simulink model "evaluate_original_controller"  (R2020b)
settings: Solver=VariableStepAuto  StartTime=0.0  StopTime=100  RelTol=1e-3
settings Model: Creator=sharm  LastModifiedBy=Abhijit

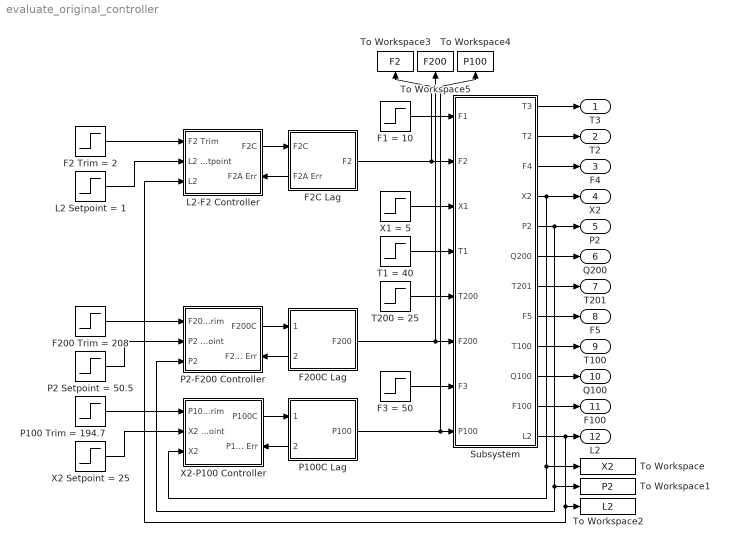
== system evaluate_original_controller ==
  F1 = 10 : Step  Time=0  After=10  SampleTime=0
  F2 Trim = 2 : Step  Time=0  After=2  SampleTime=0
  F200 Trim = 208 : Step  Time=0  After=208  SampleTime=0
  F200C Lag : Subsystem
      settings: PortSchema="{\"entries\":[{\"content\":{\"sides\":[{\"content\":{\"connectorIds\":[\"In1\",\"Out2\"]},\"type\":\"ConnectorPlacement.EquallySpacedRectSide\",\"uuid\":\"1c3b5bbe-eb64-4cf8-b304-9bf07220404b\"},{\"content\":{\"connectorIds\":[\"Out1\"],\"side\":\"RIGHT\"},\"type\":\"ConnectorPlacement.EquallySpacedRectSide\",\"uuid\":\"6c2af0ff-ea38-462b-984a-3066c6908657\"},{\"content\":{\"connectorIds\":[],\"side\":\"TOP\"},\"type\":\"ConnectorPlacement.EquallySpacedRectSide\",\"uuid\":\"8a7c128d-c093-40ae-be05-769f76d364e8\"},{\"content\":{\"connectorIds\":[],\"side\":\"HIDDEN\"},\"type\":\"ConnectorPlacement.EquallySpacedRectSide\",\"uuid\":\"6249208d-1a89-4983-a2d1-3ae1d70edd23\"}]},\"type\":\"ConnectorPlacement.EquallySpacedConnector\",\"uuid\":\"06c805ce-2383-4e6d-828b-e0ccee0563b2\"}],\"packageUris\":[\"http://schema.mathworks.com/mf0/Connector/R2020b\"],\"version\":\"1.0\"}"
  F2C Lag : Subsystem
      settings: PortSchema="{\"entries\":[{\"content\":{\"sides\":[{\"content\":{\"connectorIds\":[\"In1\",\"Out2\"]},\"type\":\"ConnectorPlacement.EquallySpacedRectSide\",\"uuid\":\"1c3b5bbe-eb64-4cf8-b304-9bf07220404b\"},{\"content\":{\"connectorIds\":[\"Out1\"],\"side\":\"RIGHT\"},\"type\":\"ConnectorPlacement.EquallySpacedRectSide\",\"uuid\":\"6c2af0ff-ea38-462b-984a-3066c6908657\"},{\"content\":{\"connectorIds\":[],\"side\":\"TOP\"},\"type\":\"ConnectorPlacement.EquallySpacedRectSide\",\"uuid\":\"8a7c128d-c093-40ae-be05-769f76d364e8\"},{\"content\":{\"connectorIds\":[],\"side\":\"HIDDEN\"},\"type\":\"ConnectorPlacement.EquallySpacedRectSide\",\"uuid\":\"6249208d-1a89-4983-a2d1-3ae1d70edd23\"}]},\"type\":\"ConnectorPlacement.EquallySpacedConnector\",\"uuid\":\"06c805ce-2383-4e6d-828b-e0ccee0563b2\"}],\"packageUris\":[\"http://schema.mathworks.com/mf0/Connector/R2020b\"],\"version\":\"1.0\"}"
  F3 = 50 : Step  Time=0  After=50  SampleTime=0
  L2 Setpoint = 1 : Step  Time=0  SampleTime=0
  L2-F2 Controller : Subsystem
      settings: PortSchema="{\"entries\":[{\"content\":{\"sides\":[{\"content\":{\"connectorIds\":[\"In1\",\"In2\",\"In3\"]},\"type\":\"ConnectorPlacement.EquallySpacedRectSide\",\"uuid\":\"ef4d4ad5-d901-40f4-ab80-7b76a95becde\"},{\"content\":{\"connectorIds\":[\"Out1\",\"In4\"],\"side\":\"RIGHT\"},\"type\":\"ConnectorPlacement.EquallySpacedRectSide\",\"uuid\":\"2e3077cf-f85a-4001-bdaf-12bb693cb162\"},{\"content\":{\"connectorIds\":[],\"side\":\"TOP\"},\"type\":\"ConnectorPlacement.EquallySpacedRectSide\",\"uuid\":\"9371a95a-1f33-4289-96cf-45c2d57bb552\"},{\"content\":{\"connectorIds\":[],\"side\":\"HIDDEN\"},\"type\":\"ConnectorPlacement.EquallySpacedRectSide\",\"uuid\":\"48f9f8fb-fea7-44ca-a8f8-23ec64a6d384\"}]},\"type\":\"ConnectorPlacement.EquallySpacedConnector\",\"uuid\":\"95306fdf-8f22-41f0-a056-501cc3b95527\"}],\"packageUris\":[\"http://schema.mathworks.com/mf0/Connector/R2020b\"],\"version\":\"1.0\"}"
  P100 Trim = 194.7 : Step  Time=0  After=194.7  SampleTime=0
  P100C Lag : Subsystem
      settings: PortSchema="{\"entries\":[{\"content\":{\"sides\":[{\"content\":{\"connectorIds\":[\"In1\",\"Out2\"]},\"type\":\"ConnectorPlacement.EquallySpacedRectSide\",\"uuid\":\"1c3b5bbe-eb64-4cf8-b304-9bf07220404b\"},{\"content\":{\"connectorIds\":[\"Out1\"],\"side\":\"RIGHT\"},\"type\":\"ConnectorPlacement.EquallySpacedRectSide\",\"uuid\":\"6c2af0ff-ea38-462b-984a-3066c6908657\"},{\"content\":{\"connectorIds\":[],\"side\":\"TOP\"},\"type\":\"ConnectorPlacement.EquallySpacedRectSide\",\"uuid\":\"8a7c128d-c093-40ae-be05-769f76d364e8\"},{\"content\":{\"connectorIds\":[],\"side\":\"HIDDEN\"},\"type\":\"ConnectorPlacement.EquallySpacedRectSide\",\"uuid\":\"6249208d-1a89-4983-a2d1-3ae1d70edd23\"}]},\"type\":\"ConnectorPlacement.EquallySpacedConnector\",\"uuid\":\"06c805ce-2383-4e6d-828b-e0ccee0563b2\"}],\"packageUris\":[\"http://schema.mathworks.com/mf0/Connector/R2020b\"],\"version\":\"1.0\"}"
  P2 Setpoint = 50.5 : Step  Time=0  After=50.5  SampleTime=0
  P2-F200 Controller : Subsystem
      settings: PortSchema="{\"entries\":[{\"content\":{\"sides\":[{\"content\":{\"connectorIds\":[\"In1\",\"In2\",\"In3\"]},\"type\":\"ConnectorPlacement.EquallySpacedRectSide\",\"uuid\":\"efbfbbac-d1e8-4a8e-b8ab-62373299654b\"},{\"content\":{\"connectorIds\":[\"Out1\",\"In4\"],\"side\":\"RIGHT\"},\"type\":\"ConnectorPlacement.EquallySpacedRectSide\",\"uuid\":\"c58e02ed-8699-419e-a739-83aeea4730ec\"},{\"content\":{\"connectorIds\":[],\"side\":\"TOP\"},\"type\":\"ConnectorPlacement.EquallySpacedRectSide\",\"uuid\":\"6be78c43-8237-4941-bb5c-cd018c1dcd72\"},{\"content\":{\"connectorIds\":[],\"side\":\"HIDDEN\"},\"type\":\"ConnectorPlacement.EquallySpacedRectSide\",\"uuid\":\"857e6460-9b7a-4c8b-b076-9e161e4e69bc\"}]},\"type\":\"ConnectorPlacement.EquallySpacedConnector\",\"uuid\":\"c2581144-7ad0-4f3d-846a-09b725ec330e\"}],\"packageUris\":[\"http://schema.mathworks.com/mf0/Connector/R2020b\"],\"version\":\"1.0\"}"
  Subsystem : Subsystem
  T1 = 40 : Step  Time=0  After=40  SampleTime=0
  T200 = 25 : Step  Time=0  After=25  SampleTime=0
  To Workspace : ToWorkspace  VariableName=X2  SaveFormat=Timeseries  SampleTime=-1
  To Workspace1 : ToWorkspace  VariableName=P2  SaveFormat=Timeseries  SampleTime=-1
  To Workspace2 : ToWorkspace  VariableName=L2  SaveFormat=Timeseries  SampleTime=-1
  To Workspace3 : ToWorkspace  VariableName=F2  SaveFormat=Timeseries  SampleTime=-1
  To Workspace4 : ToWorkspace  VariableName=P100  SaveFormat=Timeseries  SampleTime=-1
  To Workspace5 : ToWorkspace  VariableName=F200  SaveFormat=Timeseries  SampleTime=-1
  X1 = 5 : Step  Time=0  After=5  SampleTime=0
  X2 Setpoint = 25 : Step  Time=0  After=25  SampleTime=0
  X2-P100 Controller : Subsystem
      settings: PortSchema="{\"entries\":[{\"content\":{\"sides\":[{\"content\":{\"connectorIds\":[\"In1\",\"In2\",\"In3\"]},\"type\":\"ConnectorPlacement.EquallySpacedRectSide\",\"uuid\":\"5176dffd-dac1-4f9a-92a2-c3fec1393752\"},{\"content\":{\"connectorIds\":[\"Out1\",\"In4\"],\"side\":\"RIGHT\"},\"type\":\"ConnectorPlacement.EquallySpacedRectSide\",\"uuid\":\"ca0c7e9c-49dd-444e-80c7-5413a8e537a6\"},{\"content\":{\"connectorIds\":[],\"side\":\"TOP\"},\"type\":\"ConnectorPlacement.EquallySpacedRectSide\",\"uuid\":\"a41274ea-81fe-4467-9d67-a42c6c088fa1\"},{\"content\":{\"connectorIds\":[],\"side\":\"HIDDEN\"},\"type\":\"ConnectorPlacement.EquallySpacedRectSide\",\"uuid\":\"a4d67f8d-295f-4f62-a506-6c78b119ab3d\"}]},\"type\":\"ConnectorPlacement.EquallySpacedConnector\",\"uuid\":\"c27aa63c-44fb-4ea2-acae-9f89fa1a7cde\"}],\"packageUris\":[\"http://schema.mathworks.com/mf0/Connector/R2020b\"],\"version\":\"1.0\"}"
  T3 : Outport
  T2 : Outport  Port=2
  F4 : Outport  Port=3
  X2 : Outport  Port=4
  P2 : Outport  Port=5
  Q200 : Outport  Port=6
  T201 : Outport  Port=7
  F5 : Outport  Port=8
  T100 : Outport  Port=9
  Q100 : Outport  Port=10
  F100 : Outport  Port=11
  L2 : Outport  Port=12
  wires:
  F1 = 10/1 -> Subsystem/1(F1)
  X1 = 5/1 -> Subsystem/3(X1)
  T1 = 40/1 -> Subsystem/4(T1)
  T200 = 25/1 -> Subsystem/5(T200)
  F3 = 50/1 -> Subsystem/7(F3)
  Subsystem/1(T3) -> T3/1
  Subsystem/2(T2) -> T2/1
  Subsystem/3(F4) -> F4/1
  Subsystem/4(X2) -> X2-P100 Controller/3(X2), To Workspace/1, X2/1
  Subsystem/5(P2) -> P2/1, To Workspace1/1, P2-F200 Controller/3(P2)
  Subsystem/6(Q200) -> Q200/1
  Subsystem/7(T201) -> T201/1
  Subsystem/8(F5) -> F5/1
  Subsystem/9(T100) -> T100/1
  Subsystem/10(Q100) -> Q100/1
  Subsystem/11(F100) -> F100/1
  Subsystem/12(L2) -> L2/1, To Workspace2/1, L2-F2 Controller/3(L2)
  X2-P100 Controller/1(P100C) -> P100C Lag/1(P100C)
  P100C Lag/2(P100A Err) -> X2-P100 Controller/4(P100A Err)
  F200C Lag/2(F200A Err) -> P2-F200 Controller/4(F200A Err)
  P2-F200 Controller/1(F200C) -> F200C Lag/1(F200C)
  L2-F2 Controller/1(F2C) -> F2C Lag/1(F2C)
  F2C Lag/2(F2A Err) -> L2-F2 Controller/4(F2A Err)
  F200C Lag/1(F200) -> To Workspace5/1, Subsystem/6(F200)
  P100C Lag/1(P100) -> To Workspace4/1, Subsystem/8(P100)
  F2C Lag/1(F2) -> To Workspace3/1, Subsystem/2(F2)
  P2 Setpoint = 50.5/1 -> P2-F200 Controller/2(P2 Setpoint)
  L2 Setpoint = 1/1 -> L2-F2 Controller/2(L2 Setpoint)
  X2 Setpoint = 25/1 -> X2-P100 Controller/2(X2 Setpoint)
  P100 Trim = 194.7/1 -> X2-P100 Controller/1(P100 Trim)
  F2 Trim = 2/1 -> L2-F2 Controller/1(F2 Trim)
  F200 Trim = 208/1 -> P2-F200 Controller/1(F200 Trim)

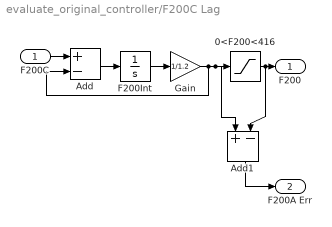
== system evaluate_original_controller/F200C Lag ==
  F200C : Inport
  0<F200<416 : Saturate  UpperLimit=416  LowerLimit=0
  Add : Sum  Inputs=+-
  Add1 : Sum  Inputs=+-
  F200Int : Integrator  InitialCondition=208
  Gain : Gain  Gain=1/1.2
  F200 : Outport
  F200A Err : Outport  Port=2
  wires:
  Gain/1 -> Add/2, Add1/1, 0<F200<416/1
  Add/1 -> F200Int/1
  F200Int/1 -> Gain/1
  F200C/1 -> Add/1
  0<F200<416/1 -> Add1/2, F200/1
  Add1/1 -> F200A Err/1

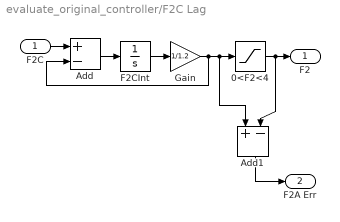
== system evaluate_original_controller/F2C Lag ==
  F2C : Inport
  0<F2<4 : Saturate  UpperLimit=4  LowerLimit=0
  Add : Sum  Inputs=+-
  Add1 : Sum  Inputs=+-
  F2CInt : Integrator  InitialCondition=2
  Gain : Gain  Gain=1/1.2
  F2 : Outport
  F2A Err : Outport  Port=2
  wires:
  Gain/1 -> Add/2, Add1/1, 0<F2<4/1
  Add/1 -> F2CInt/1
  F2CInt/1 -> Gain/1
  F2C/1 -> Add/1
  0<F2<4/1 -> Add1/2, F2/1
  Add1/1 -> F2A Err/1

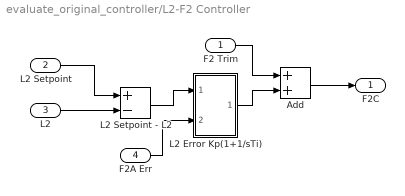
== system evaluate_original_controller/L2-F2 Controller ==
  F2 Trim : Inport
  L2 Setpoint : Inport  Port=2
  L2 : Inport  Port=3
  F2A Err : Inport  Port=4
  Add : Sum
  L2 Error Kp(1+1/sTi) : Subsystem
  L2 Setpoint - L2 : Sum  Inputs=+-
  F2C : Outport
  wires:
  L2 Setpoint/1 -> L2 Setpoint - L2/1
  F2 Trim/1 -> Add/1
  L2/1 -> L2 Setpoint - L2/2
  L2 Error Kp(1+1/sTi)/1(dF2C) -> Add/2
  L2 Setpoint - L2/1 -> L2 Error Kp(1+1/sTi)/1(F2 Err)
  Add/1 -> F2C/1
  F2A Err/1 -> L2 Error Kp(1+1/sTi)/2(F2A Err)

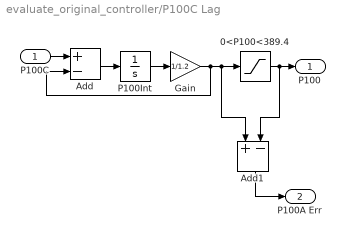
== system evaluate_original_controller/P100C Lag ==
  P100C : Inport
  0<P100<389.4 : Saturate  UpperLimit=389.4  LowerLimit=0
  Add : Sum  Inputs=+-
  Add1 : Sum  Inputs=+-
  Gain : Gain  Gain=1/1.2
  P100Int : Integrator  InitialCondition=194.7
  P100 : Outport
  P100A Err : Outport  Port=2
  wires:
  Gain/1 -> Add/2, 0<P100<389.4/1, Add1/1
  Add/1 -> P100Int/1
  P100Int/1 -> Gain/1
  P100C/1 -> Add/1
  0<P100<389.4/1 -> Add1/2, P100/1
  Add1/1 -> P100A Err/1

== system evaluate_original_controller/P2-F200 Controller ==
  F200 Trim : Inport
  P2 Setpoint : Inport  Port=2
  P2 : Inport  Port=3
  F200A Err : Inport  Port=4
  Add : Sum
  P2 Error Kp(1+1/sTi) : Subsystem
  P2 Setpoint - P2 : Sum  Inputs=+-
  F200C : Outport
  wires:
  P2 Setpoint/1 -> P2 Setpoint - P2/1
  F200 Trim/1 -> Add/1
  Add/1 -> F200C/1
  P2/1 -> P2 Setpoint - P2/2
  P2 Error Kp(1+1/sTi)/1(dF200C) -> Add/2
  P2 Setpoint - P2/1 -> P2 Error Kp(1+1/sTi)/1(P2 Err)
  F200A Err/1 -> P2 Error Kp(1+1/sTi)/2(F200A Err)

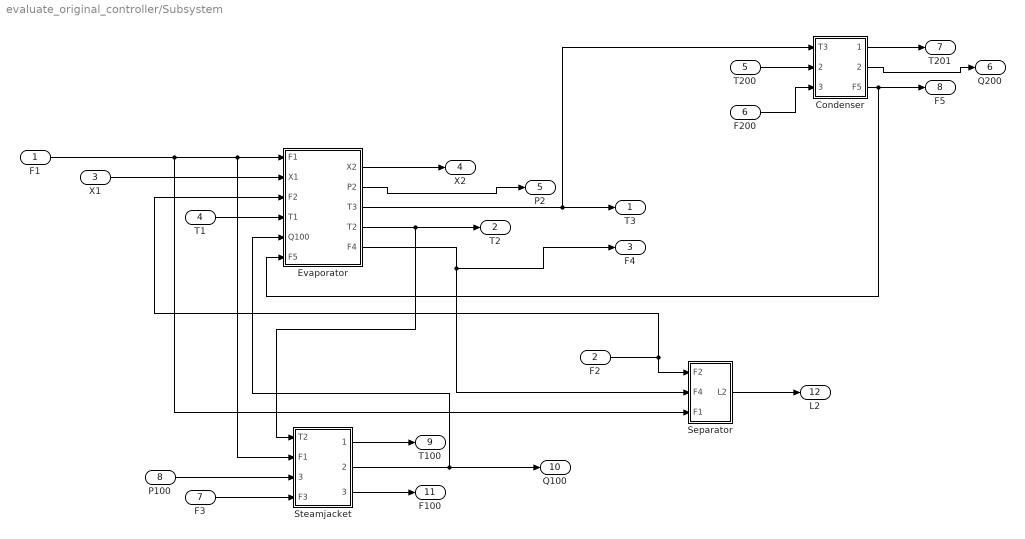
== system evaluate_original_controller/Subsystem ==
  F1 : Inport
  F2 : Inport  Port=2
  X1 : Inport  Port=3
  T1 : Inport  Port=4
  T200 : Inport  Port=5
  F200 : Inport  Port=6
  F3 : Inport  Port=7
  P100 : Inport  Port=8
  Condenser : Subsystem
  Evaporator : Subsystem
  Separator : Subsystem
  Steamjacket : Subsystem
  T3 : Outport
  T2 : Outport  Port=2
  F4 : Outport  Port=3
  X2 : Outport  Port=4
  P2 : Outport  Port=5
  Q200 : Outport  Port=6
  T201 : Outport  Port=7
  F5 : Outport  Port=8
  T100 : Outport  Port=9
  Q100 : Outport  Port=10
  F100 : Outport  Port=11
  L2 : Outport  Port=12
  wires:
  X1/1 -> Evaporator/2(X1)
  Condenser/3(F5) -> F5/1, Evaporator/6(F5)
  T200/1 -> Condenser/2(T200)
  Condenser/1(T201) -> T201/1
  Steamjacket/2(Q100) -> Q100/1, Evaporator/5(Q100)
  F1/1 -> Steamjacket/2(F1), Evaporator/1(F1), Separator/3(F1)
  Evaporator/2(P2) -> P2/1
  Evaporator/3(T3) -> T3/1, Condenser/1(T3)
  Evaporator/1(X2) -> X2/1
  F2/1 -> Evaporator/3(F2), Separator/1(F2)
  T1/1 -> Evaporator/4(T1)
  Evaporator/5(F4) -> F4/1, Separator/2(F4)
  Steamjacket/3(F100) -> F100/1
  F3/1 -> Steamjacket/4(F3)
  P100/1 -> Steamjacket/3(P100)
  Evaporator/4(T2) -> T2/1, Steamjacket/1(T2)
  Steamjacket/1(T100) -> T100/1
  Condenser/2(Q200) -> Q200/1
  F200/1 -> Condenser/3(F200)
  Separator/1(L2) -> L2/1

== system evaluate_original_controller/X2-P100 Controller ==
  P100 Trim : Inport
  X2 Setpoint : Inport  Port=2
  X2 : Inport  Port=3
  P100A Err : Inport  Port=4
  Add : Sum
  P100 Error Kp(1+1/sTi) : Subsystem
  X2 Setpoint - X2 : Sum  Inputs=+-
  P100C : Outport
  wires:
  X2 Setpoint/1 -> X2 Setpoint - X2/1
  P100 Trim/1 -> Add/1
  Add/1 -> P100C/1
  X2/1 -> X2 Setpoint - X2/2
  P100 Error Kp(1+1/sTi)/1(dP100C) -> Add/2
  X2 Setpoint - X2/1 -> P100 Error Kp(1+1/sTi)/1(X2 Err)
  P100A Err/1 -> P100 Error Kp(1+1/sTi)/2(P100A Err)

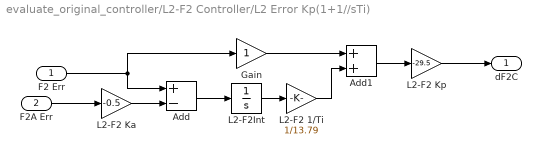
== system evaluate_original_controller/L2-F2 Controller/L2 Error Kp(1+1//sTi) ==
  F2 Err : Inport
  F2A Err : Inport  Port=2
  Add : Sum  Inputs=+-
  Add1 : Sum
  Gain : Gain
  L2-F2 1/Ti : Gain  Gain=1/13.79
  L2-F2 Ka : Gain  Gain=-0.5
  L2-F2 Kp : Gain  Gain=-29.5
  L2-F2Int : Integrator
  dF2C : Outport
  wires:
  L2-F2 1/Ti/1 -> Add1/2
  L2-F2 Kp/1 -> dF2C/1
  Add1/1 -> L2-F2 Kp/1
  Gain/1 -> Add1/1
  L2-F2Int/1 -> L2-F2 1/Ti/1
  F2 Err/1 -> Add/1, Gain/1
  F2A Err/1 -> L2-F2 Ka/1
  L2-F2 Ka/1 -> Add/2
  Add/1 -> L2-F2Int/1

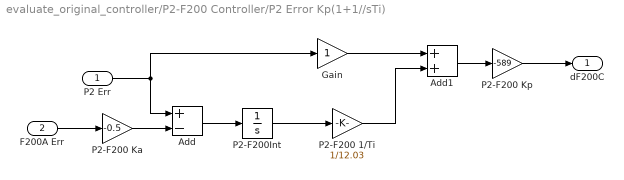
== system evaluate_original_controller/P2-F200 Controller/P2 Error Kp(1+1//sTi) ==
  P2 Err : Inport
  F200A Err : Inport  Port=2
  Add : Sum  Inputs=+-
  Add1 : Sum
  Gain : Gain
  P2-F200 1/Ti : Gain  Gain=1/12.03
  P2-F200 Ka : Gain  Gain=-0.5
  P2-F200 Kp : Gain  Gain=-589
  P2-F200Int : Integrator
  dF200C : Outport
  wires:
  P2 Err/1 -> Add/1, Gain/1
  P2-F200 Kp/1 -> dF200C/1
  Add1/1 -> P2-F200 Kp/1
  Gain/1 -> Add1/1
  P2-F200Int/1 -> P2-F200 1/Ti/1
  P2-F200 1/Ti/1 -> Add1/2
  Add/1 -> P2-F200Int/1
  F200A Err/1 -> P2-F200 Ka/1
  P2-F200 Ka/1 -> Add/2

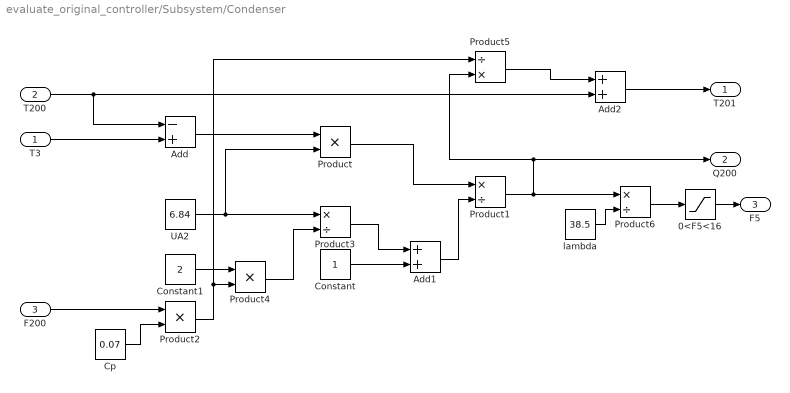
== system evaluate_original_controller/Subsystem/Condenser ==
  T3 : Inport
  T200 : Inport  Port=2
  F200 : Inport  Port=3
  0<F5<16 : Saturate  UpperLimit=16  LowerLimit=0
  Add : Sum  Inputs=-+
  Add1 : Sum
  Add2 : Sum
  Constant : Constant
  Constant1 : Constant  Value=2
  Cp : Constant  Value=0.07
  Product : Product
  Product1 : Product  Inputs=*/
  Product2 : Product
  Product3 : Product  Inputs=*/
  Product4 : Product
  Product5 : Product  Inputs=/*
  Product6 : Product  Inputs=*/
  UA2 : Constant  Value=6.84
  lambda : Constant  Value=38.5
  T201 : Outport
  Q200 : Outport  Port=2
  F5 : Outport  Port=3
  wires:
  Product1/1 -> Q200/1, Product5/2, Product6/1
  lambda/1 -> Product6/2
  Product5/1 -> Add2/1
  Constant1/1 -> Product4/1
  Product2/1 -> Product5/1, Product4/2
  Constant/1 -> Add1/2
  Add/1 -> Product/1
  Cp/1 -> Product2/2
  Product4/1 -> Product3/2
  T200/1 -> Add2/2, Add/1
  Product/1 -> Product1/1
  Add2/1 -> T201/1
  Product3/1 -> Add1/1
  UA2/1 -> Product3/1, Product/2
  T3/1 -> Add/2
  F200/1 -> Product2/1
  Add1/1 -> Product1/2
  Product6/1 -> 0<F5<16/1
  0<F5<16/1 -> F5/1

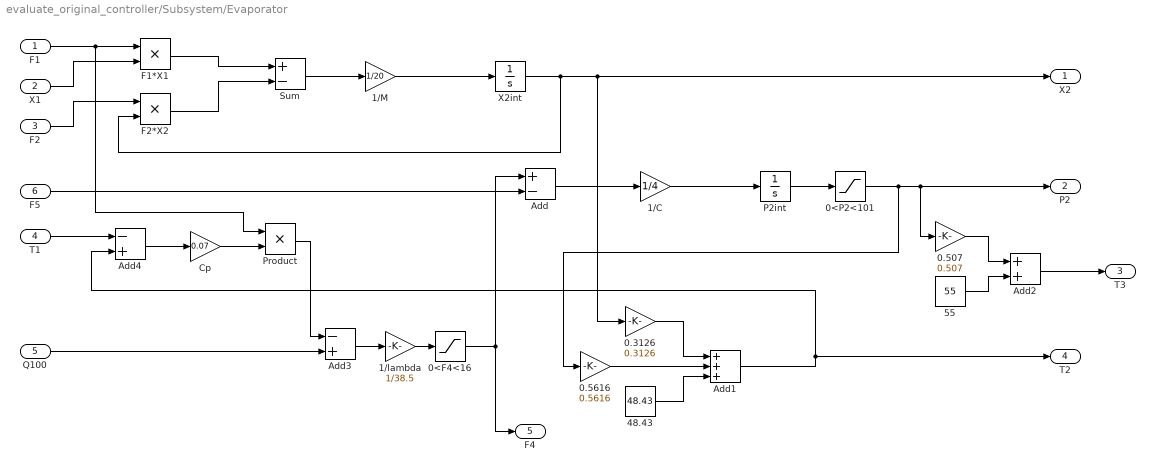
== system evaluate_original_controller/Subsystem/Evaporator ==
  F1 : Inport
  X1 : Inport  Port=2
  F2 : Inport  Port=3
  T1 : Inport  Port=4
  Q100 : Inport  Port=5
  F5 : Inport  Port=6
  0.3126 : Gain  Gain=0.3126
  0.507 : Gain  Gain=0.507
  0.5616 : Gain  Gain=0.5616
  0<F4<16 : Saturate  UpperLimit=16  LowerLimit=0
  0<P2<101 : Saturate  UpperLimit=101  LowerLimit=0
  1/C : Gain  Gain=1/4
  1/M : Gain  Gain=1/20
  1/lambda : Gain  Gain=1/38.5
  48.43 : Constant  Value=48.43
  55 : Constant  Value=55
  Add : Sum  Inputs=+-
  Add1 : Sum  Inputs=+++
  Add2 : Sum
  Add3 : Sum  Inputs=-+
  Add4 : Sum  Inputs=-+
  Cp : Gain  Gain=0.07
  F1*X1 : Product
  F2*X2 : Product
  P2int : Integrator  InitialCondition=50.5
  Product : Product
  Sum : Sum  Inputs=+-
  X2int : Integrator  InitialCondition=25
  X2 : Outport
  P2 : Outport  Port=2
  T3 : Outport  Port=3
  T2 : Outport  Port=4
  F4 : Outport  Port=5
  wires:
  Product/1 -> Add3/1
  Add4/1 -> Cp/1
  Add1/1 -> T2/1, Add4/2
  Add/1 -> 1/C/1
  F1/1 -> Product/1, F1*X1/1
  Add2/1 -> T3/1
  X2int/1 -> X2/1, 0.3126/1, F2*X2/2
  0.507/1 -> Add2/1
  Cp/1 -> Product/2
  F1*X1/1 -> Sum/1
  0.3126/1 -> Add1/1
  1/C/1 -> P2int/1
  F2/1 -> F2*X2/1
  1/M/1 -> X2int/1
  Sum/1 -> 1/M/1
  48.43/1 -> Add1/3
  F2*X2/1 -> Sum/2
  Add3/1 -> 1/lambda/1
  Q100/1 -> Add3/2
  F5/1 -> Add/2
  55/1 -> Add2/2
  0.5616/1 -> Add1/2
  T1/1 -> Add4/1
  X1/1 -> F1*X1/2
  0<F4<16/1 -> F4/1, Add/1
  1/lambda/1 -> 0<F4<16/1
  P2int/1 -> 0<P2<101/1
  0<P2<101/1 -> 0.5616/1, 0.507/1, P2/1

== system evaluate_original_controller/Subsystem/Separator ==
  F2 : Inport
  F4 : Inport  Port=2
  F1 : Inport  Port=3
  0<L2<2 : Saturate  UpperLimit=2  LowerLimit=0
  1/rhoA : Gain  Gain=1/20
  L2int : Integrator  InitialCondition=1
  Sum : Sum  Inputs=+--
  L2 : Outport
  wires:
  F4/1 -> Sum/3
  1/rhoA/1 -> L2int/1
  Sum/1 -> 1/rhoA/1
  F2/1 -> Sum/2
  F1/1 -> Sum/1
  L2int/1 -> 0<L2<2/1
  0<L2<2/1 -> L2/1

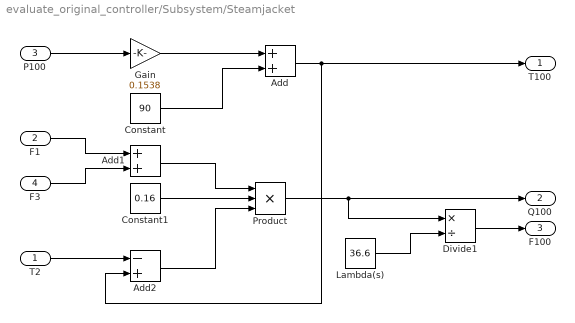
== system evaluate_original_controller/Subsystem/Steamjacket ==
  T2 : Inport
  F1 : Inport  Port=2
  P100 : Inport  Port=3
  F3 : Inport  Port=4
  Add : Sum
  Add1 : Sum
  Add2 : Sum  Inputs=-+
  Constant : Constant  Value=90
  Constant1 : Constant  Value=0.16
  Divide1 : Product  Inputs=*/
  Gain : Gain  Gain=0.1538
  Lambda(s) : Constant  Value=36.6  VectorParams1D=off
  Product : Product  Inputs=3
  T100 : Outport
  Q100 : Outport  Port=2
  F100 : Outport  Port=3
  wires:
  Add1/1 -> Product/1
  Constant1/1 -> Product/2
  Product/1 -> Q100/1, Divide1/1
  Gain/1 -> Add/1
  Add2/1 -> Product/3
  Lambda(s)/1 -> Divide1/2
  Constant/1 -> Add/2
  Add/1 -> T100/1, Add2/2
  P100/1 -> Gain/1
  T2/1 -> Add2/1
  Divide1/1 -> F100/1
  F3/1 -> Add1/2
  F1/1 -> Add1/1

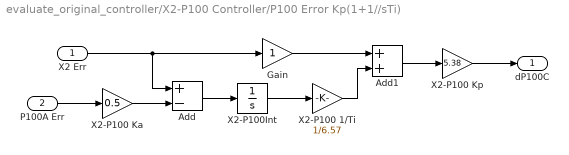
== system evaluate_original_controller/X2-P100 Controller/P100 Error Kp(1+1//sTi) ==
  X2 Err : Inport
  P100A Err : Inport  Port=2
  Add : Sum  Inputs=+-
  Add1 : Sum
  Gain : Gain
  X2-P100 1/Ti : Gain  Gain=1/6.57
  X2-P100 Ka : Gain  Gain=0.5
  X2-P100 Kp : Gain  Gain=5.38
  X2-P100Int : Integrator
  dP100C : Outport
  wires:
  X2-P100 1/Ti/1 -> Add1/2
  X2-P100 Kp/1 -> dP100C/1
  Add1/1 -> X2-P100 Kp/1
  Gain/1 -> Add1/1
  X2-P100Int/1 -> X2-P100 1/Ti/1
  P100A Err/1 -> X2-P100 Ka/1
  X2-P100 Ka/1 -> Add/2
  Add/1 -> X2-P100Int/1
  X2 Err/1 -> Gain/1, Add/1
